simulink model "gerMPC"  (Simulink 9.1)
settings: Solver=VariableStepAuto  StartTime=0.0  StopTime=40  RelTol=1e-3
libraries: Solver_SF x1, simulink x1
settings Model: Creator=MaoWenJie  LastModifiedBy=MaoWenJie
settings DataIOCC: SaveFormat=Dataset
settings OptimizationCC: LifeSpan=auto
settings DebuggingCC: UnderspecifiedInitializationDetection=Simplified  MergeDetectMultiDrivingBlocksExec=error  SFUnexpectedBacktrackingDiag=error  SFNoUnconditionalDefaultTransitionDiag=error  SFExecutionAtInitializationDiag=warning
settings HardwareCC: ProdBitPerPointer=64  ProdBitPerSizeT=64  ProdBitPerPtrDiffT=64  ProdLargestAtomicFloat=Float  ProdIntDivRoundTo=Zero  ProdEndianess=LittleEndian  ProdWordSize=64  ProdHWDeviceType=Intel->x86-64 (Windows64)
settings ModelReferenceCC: PropagateSignalLabelsOutOfModel=on
settings CodeAppCC: StateflowObjectComments=off
settings GRTTargetCC: TargetLangStandard=C99 (ISO)  CombineOutputUpdateFcns=on  GRTInterface=off
settings ConfigComp: CovMetricSettings=dwe  CovHtmlReporting=off  CovSaveCumulativeToWorkspaceVar=off  CovSaveSingleToWorkspaceVar=off  CovExternalEMLEnable=on

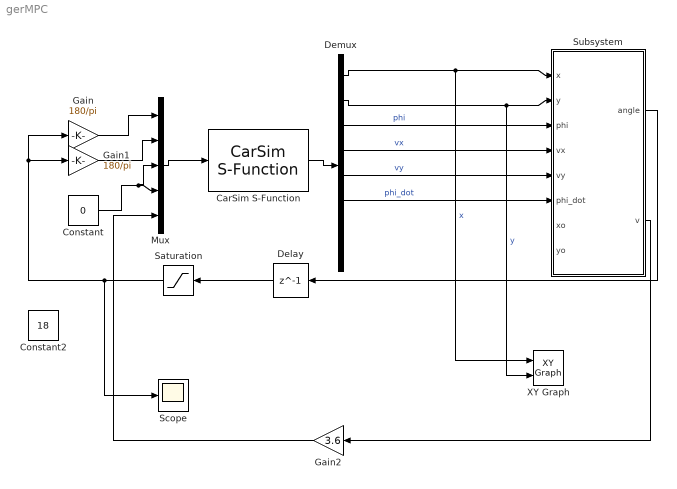
== system gerMPC ==
  CarSim S-Function : Solver_SF/CarSim S-Function  Priority=1  SIMFILE=simfile.sim
  Constant : Constant  Value=0
  Constant2 : Constant  Value=18
  Delay : Delay  DelayLength=1  UseCircularBuffer=on
  Demux : Demux  Outputs=8
  Gain : Gain  Gain=180/pi
  Gain1 : Gain  Gain=180/pi
  Gain2 : Gain  Gain=3.6
  Mux : Mux  Inputs=5
  Saturation : Saturate  UpperLimit=1.2  LowerLimit=-1.2
  Scope : Scope
  Subsystem : Subsystem
  XY Graph : simulink/Sinks/XY Graph  xmin=0  xmax=80  ymin=-50  ymax=50  st=-1
  wires:
  Subsystem/1(angle) -> Delay/1
  Demux/6 -> Subsystem/6(phi_dot)  "phi_dot"
  Mux/1 -> CarSim S-Function/1
  Delay/1 -> Saturation/1
  Demux/3 -> Subsystem/3(phi)  "phi"
  Demux/2 -> XY Graph/2, Subsystem/2(y)  "y"
  Saturation/1 -> Scope/1, Gain1/1, Gain/1
  Demux/1 -> XY Graph/1, Subsystem/1(x)  "x"
  Demux/5 -> Subsystem/5(vy)  "vy"
  CarSim S-Function/1 -> Demux/1
  Demux/4 -> Subsystem/4(vx)  "vx"
  Gain/1 -> Mux/1
  Gain1/1 -> Mux/2
  Constant/1 -> Mux/3, Mux/4
  Subsystem/2(v) -> Gain2/1
  Gain2/1 -> Mux/5

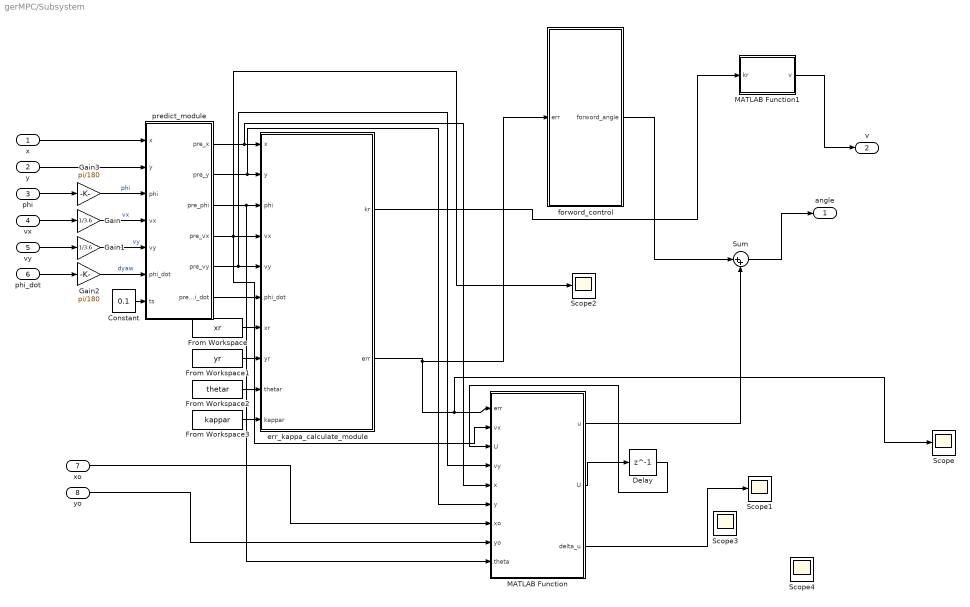
== system gerMPC/Subsystem ==
  x : Inport
  y : Inport  Port=2
  phi : Inport  Port=3
  vx : Inport  Port=4
  vy : Inport  Port=5
  phi_dot : Inport  Port=6
  xo : Inport  Port=7
  yo : Inport  Port=8
  Constant : Constant  Value=0.1
  Delay : Delay  DelayLength=1  InitialCondition=0
  From Workspace : FromWorkspace  VariableName=xr  SampleTime=0
  From Workspace1 : FromWorkspace  VariableName=yr  SampleTime=0
  From Workspace2 : FromWorkspace  VariableName=thetar  SampleTime=0
  From Workspace3 : FromWorkspace  VariableName=kappar  SampleTime=0
  Gain : Gain  Gain=1/3.6
  Gain1 : Gain  Gain=1/3.6
  Gain2 : Gain  Gain=pi/180
  Gain3 : Gain  Gain=pi/180
  MATLAB Function : MATLAB Function  InitFcn=U = 0;err = [0;0;0;0];vx = 0;val = 0;  TreatAsAtomicUnit=on
  MATLAB Function1 : MATLAB Function  TreatAsAtomicUnit=on
  Scope{,1..4} (5 alike) : Scope
  Sum : Sum  Inputs=|++
  err_kappa_calculate_module : MATLAB Function  TreatAsAtomicUnit=on
  forword_control : MATLAB Function  TreatAsAtomicUnit=on
  predict_module : MATLAB Function  TreatAsAtomicUnit=on
  angle : Outport
  v : Outport  Port=2
  wires:
  Gain1/1 -> predict_module/5(vy)  "vy"
  x/1 -> predict_module/1(x)
  phi_dot/1 -> Gain2/1
  predict_module/2(pre_y) -> MATLAB Function/6(y), err_kappa_calculate_module/2(y)
  vx/1 -> Gain/1
  predict_module/4(pre_vx) -> Scope2/1, MATLAB Function/2(vx), err_kappa_calculate_module/4(vx)
  Gain2/1 -> predict_module/6(phi_dot)  "dyaw"
  Sum/1 -> angle/1
  phi/1 -> Gain3/1
  From Workspace2/1 -> err_kappa_calculate_module/9(thetar)
  Gain/1 -> predict_module/4(vx)  "vx"
  y/1 -> predict_module/2(y)
  Gain3/1 -> predict_module/3(phi)  "phi"
  From Workspace3/1 -> err_kappa_calculate_module/10(kappar)
  Constant/1 -> predict_module/7(ts)
  From Workspace1/1 -> err_kappa_calculate_module/8(yr)
  predict_module/1(pre_x) -> MATLAB Function/5(x), err_kappa_calculate_module/1(x)
  predict_module/5(pre_vy) -> MATLAB Function/4(vy), err_kappa_calculate_module/5(vy)
  vy/1 -> Gain1/1
  From Workspace/1 -> err_kappa_calculate_module/7(xr)
  predict_module/6(pre_phi_dot) -> err_kappa_calculate_module/6(phi_dot)
  predict_module/3(pre_phi) -> MATLAB Function/9(theta), err_kappa_calculate_module/3(phi)
  err_kappa_calculate_module/2(err) -> forword_control/1(err), Scope/1, MATLAB Function/1(err)
  MATLAB Function/1(u) -> Sum/2
  forword_control/1(forword_angle) -> Sum/1
  MATLAB Function/2(U) -> Delay/1
  Delay/1 -> MATLAB Function/3("U ")
  MATLAB Function/3(delta_u) -> Scope1/1
  xo/1 -> MATLAB Function/7(xo)
  yo/1 -> MATLAB Function/8(yo)
  err_kappa_calculate_module/1(kr) -> MATLAB Function1/1(kr)
  MATLAB Function1/1(v) -> v/1

== matlab function Subsystem/err_kappa_calculate_module ==
  data: x input double; kr output double; y input double; phi input double; vx input double; vy input double; phi_dot input double; xr input double; yr input double; thetar input double; kappar input double; err output double
function [kr,err] = fcn(x,y,phi,vx,vy,phi_dot,xr,yr,thetar,kappar)
    n=length(xr);
    d_min=(x-xr(1))^2+(y-yr(1))^2;
    min=1;
    for i=1:n
        d=(x-xr(i))^2+(y-yr(i))^2;
        if d<d_min
            d_min=d;
            min=i;
        end
    end
    dmin=min;
    tor=[cos(thetar(dmin));sin(thetar(dmin))];
    nor=[-sin(thetar(dmin));cos(thetar(dmin))];
    d_err=[x-xr(dmin);y-yr(dmin)];
    ed=nor'*d_err;
    es=tor'*d_err;
    %projection_point_thetar=thetar(dmin);%apollo
    projection_point_thetar=thetar(dmin)+kappar(dmin)*es;
    ed_dot=vy*cos(phi-projection_point_thetar)+vx*sin(phi-projection_point_thetar);
    %%%%%%%%%
    ephi=sin(phi-projection_point_thetar);
    %%%%%%%%%
    s_dot=vx*cos(phi-projection_point_thetar)-vy*sin(phi-projection_point_thetar);
    s_dot=s_dot/(1-kappar(dmin)*ed);
    ephi_dot=phi_dot-kappar(dmin)*s_dot;
    kr=kappar(dmin);
    err=[ed;ed_dot;ephi;ephi_dot];
    
    
    
    
    
    
    
    
    
    
    
    


end

== matlab function Subsystem/predict_module ==
  data: x input double; pre_x output double; y input double; phi input double; vx input double; vy input double; phi_dot input double; ts input double; pre_y output double; pre_phi output double; pre_vx output double; pre_vy output double; pre_phi_dot output double
function [pre_x,pre_y,pre_phi,pre_vx,pre_vy,pre_phi_dot] = fcn(x,y,phi,vx,vy,phi_dot,ts)
    pre_x=x+vx*ts*cos(phi)-vy*ts*sin(phi);
    pre_y=y+vy*ts*cos(phi)+vx*ts*sin(phi);
    pre_phi=phi+phi_dot*ts;
    pre_vx=vx;
    pre_vy=vy;
    pre_phi_dot=phi_dot;
end

== matlab function Subsystem/MATLAB Function1 ==
  data: kr input double; v output double
function v = Control_v(kr)
% if kr == 0
%     v = 5;
% else
%     v = min(0.5*sqrt(0.9*9.8/abs(kr)),5);
v= 10;
end

== matlab function Subsystem/forword_control ==
  data: err input double; forword_angle output double
function forword_angle = fcn(err)
    %forword_angle=(1.6473+0.0069*vx^2)*kr;
    %forword_angle = 0;
    kp = 0.1
    forword_angle = -kp*err(1);
end

== matlab function Subsystem/MATLAB Function ==
  data: err input double; u output double; vx input double; U input double; U output double; delta_u output double; vy input double; x input double; y input double; xo input double; yo input double; theta input double
function [u,U,delta_u]   = ...
    MPC_control(err,vx,U,vy,x,y,xo,yo,theta) 
coder.extrinsic('dlqr');
coder.extrinsic('optimoptions');
coder.extrinsic('quadprog');
% U = 0;
% err = zeros(4,1);
% vx = 5;
cf=-110000;
cr=cf;
m=1412;
Iz=1536.7;
a=1.015;
b=2.910-1.015;
T = 0.01;
Nx=4;%状态量的个数
Nu =1;%控制量的个数
Np=4;%预测步长6
Nc=3;%控制步长
Row=10;%松弛因子
Q=100*eye(Nx*Np,Nx*Np);    
R=eye(Nc*Nu);
g=[0,1,0,0;
        0,(cf+cr)/(m*vx),-(cf+cr)/m,(a*cf-b*cr)/(m*vx);
        0,0,0,1;
        0,(a*cf-b*cr)/(Iz*vx),-(a*cf-b*cr)/Iz,(a*a*cf+b*b*cr)/(Iz*vx)];
h=[0;
    -cf/m;
    0;
    -a*cf/Iz];
a_ = g*T+eye(Nx);
b_ = h*T;
a_ = a_/10;
b_ = b_/10;
C = [1 0 0 0 0;0 1 0 0 0;0 0 1 0 0; 0 0 0 1 0];
    A = zeros(Nu+Nx,Nu+Nx);
    A(1:Nx,1:Nx)=a_;
    A(1:Nx,Nx+1:Nx+Nu)=b_;
    A(Nx+1:Nx+Nu,Nx+1:Nx+Nu) = eye(Nu);
    B = ones(Nx+Nu,Nu);
    B(1:Nx,:)=b_;
    B(Nx+1:Nx+Nu,:)=eye(Nu);
    Px = zeros(Nx*Np,Nx+Nu);
    Hx = zeros(Nx*Np,Nu*Nc);
    for j=1:1:Np
        Px(1+(j-1)*Nx:j*Nx,:)=C*A^j;
        for k=1:1:Nc
            if k<=j
                Hx(1+(j-1)*Nx:j*Nx,k)=C*A^(j-k)*B;
            else 
                Hx(1+(j-1)*Nx:j*Nx,k)=zeros(Nx,Nu);
            end
        end
    end
    kesi = [err;U];
    H=[Hx'*Q*Hx+R,zeros(Nu*Nc,1);
        zeros(1,Nu*Nc),Row];
    H=(H'+H)/2;
    f=[2*kesi'*Px'*Q*Hx,0];
    
 %% 以下为约束生成区域
 %不等式约束
    A_t=zeros(Nc,Nc);%见falcone论文 P181
    for p=1:1:Nc
        for q=1:1:Nc
            if q<=p 
                A_t(p,q)=1;
            else 
                A_t(p,q)=0;
            end
        end 
    end 
    A_I=A_t;%对应于falcone论文约束处理的矩阵A,求克罗内克积
    Ut=ones(Nc,1)*U;%此处感觉论文里的克罗内科积有问题,暂时交换顺序
    umin=-0.64;%维数与控制变量的个数相同
    umax=0.64;
    delta_umin = -0.64;
    delta_umax = 0.64;
    delta_Umin=ones(Nc,1)*delta_umin;
    delta_Umax=ones(Nc,1)*delta_umax;
    Umin=ones(Nc,1)*umin;
    Umax=ones(Nc,1)*umax;
    M = 10;
    %--------------my code----------------------
%     Hy = zeros(Np,Nx*Np);
%     for i = 1:Np
%         Hy(i,4*i-3)=1;
%     end
%     Ymin = -3*ones(Np,1);
%     Ymax = 3*zeros(Np,1);
    %-------------------------------------------
    
    %--------------my code----------------------
%    d = sqrt((x-xo)^2+(y-yo)^2);
%    sin_phi = (y-yo)/d;
%    cos_phi = (x-xo)/d;
%    if sin_phi>=0 && cos_phi>=0
%        phi = asin((y-yo)/d);
%    elseif sin_phi>0 && cos_phi<0
%        phi = pi - asin((y-yo)/d);
%    elseif sin_phi<0 && cos_phi<0
%        phi = -1*pi + asin((y-yo)/d);
%    else
%        phi = -1* asin((y-yo)/d);
%    end
%    
%    alaph = -2;
%    v_cbf = sqrt(vx*vx+vy*vy);
%    C_cbf = -0.5*alaph*d*d;
%    A_cbf = v_cbf*(x-xo);
%    B_cbf = v_cbf*(y-yo);
%    D_cbf = C_cbf/sqrt(A_cbf*A_cbf+B_cbf*B_cbf);
%    
%    u_cbf_min = -pi;
%    u_cbf_max = pi;
%    down = -inf;
%    up = inf;
%    if D_cbf >= -1
%       k_cbf = floor((phi+theta-pi/2)/(2*pi));
%       phi = phi - 2*k_cbf;
%       a2_cbf = asin(D_cbf);
%       a1_cbf = -1*a2_cbf -pi + 2*pi;
%       
%       down = a2_cbf - phi - theta;
%       up =  a1_cbf - phi - theta;
      
%       while down < u_cbf_min
%           down = down + 2*pi;
%       end
%       
%       while down > u_cbf_max
%           down = down - 2*pi;
%       end
%       
%       while up < u_cbf_min
%           up = up + 2*pi;
%       end
%       
%       while up > u_cbf_max
%           up = up - 2*pi;
%       end

%    end
       
  
    %--------------------------------------------
%     A_cons=[A_I zeros(Nu*Nc,1);-A_I zeros(Nu*Nc,1);Hy*Hx zeros(Np,1);-Hy*Hx zeros(Np,1)];
%     b_cons=[Umax-Ut;-Umin+Ut;Ymax-Hy*Px*kesi;-Ymin+Hy*Px*kesi];
    A_cons=[A_I zeros(Nu*Nc,1);-A_I zeros(Nu*Nc,1)];
    b_cons=[Umax-Ut;-Umin+Ut];
   % 状态量约束
%     delta_Umin(1) = max(down-U,delta_umin);
%     delta_Umax(1) = min(up-U,delta_umax);
    lb=[delta_Umin;0];%（求解方程）状态量下界，包含控制时域内控制增量和松弛因子
    ub=[delta_Umax;M];%（求解方程）状态量上界，包含控制时域内控制增量和松弛因子
    %% 开始求解过程
    delta_u = 0;
    exitflag = 0;
    X0=zeros(Nu*Nc+1,1);
    options = optimoptions('quadprog','Display','iter','MaxIterations',100,'TolFun',1e-16);
    [X,fval,exitflag]=quadprog(H,f,A_cons,b_cons,[],[],lb,ub,X0,options);
    %% 计算输出
    if exitflag==-2
    delta_u=randn(1)*0.001;
    else
    delta_u=X(1);
    end
    u = U+delta_u;
    U = u;
end
